simulink model "dual_quaternion_equation_of_motion_1"  (R2016a)
settings: Solver=ode45  StartTime=0.0  StopTime=10.0  MaxStep=0.2  RelTol=1e-3
InitFcn:
  | addpath('..');
settings Model: Creator=AkhramovichSA  LastModifiedBy=AkhramovichSA

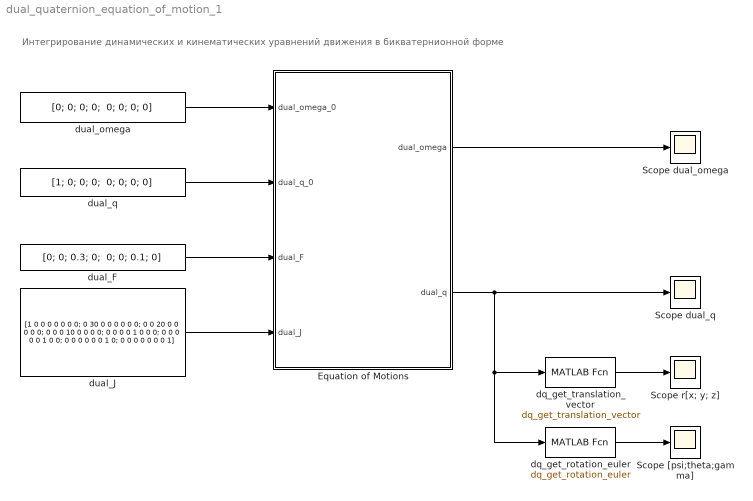
== system dual_quaternion_equation_of_motion_1 ==
  note: Интегрирование динамических и кинематических уравнений движения в бикватернионной форме
  Equation of Motions : Subsystem
  Scope [psi;theta;gamma] : Scope
  Scope dual_omega : Scope
  Scope dual_q : Scope
  Scope r[x; y; z] : Scope
  dq_get_rotation_euler : MATLABFcn  Description=aa  MATLABFcn=dq_get_rotation_euler
  dq_get_translation_vector : MATLABFcn  MATLABFcn=dq_get_translation_vector
  dual_F : Constant  Value="[0; 0; 0.3; 0;  0; 0; 0.1; 0]"  VectorParams1D=off
  dual_J : Constant  Value=[1 0 0 0 0 0 0 0; 0 30 0 0 0 0 0 0; 0 0 20 0 0 0 0 0; 0 0 0 10 0 0 0 0; 0 0 0 0 1 0 0 0; 0 0 0 0 0 1 0 0; 0 0 0 0 0 0 1 0; 0 0 0 0 0 0 0 1]  VectorParams1D=off
  dual_omega : Constant  Value="[0; 0; 0; 0;  0; 0; 0; 0]"  VectorParams1D=off
  dual_q : Constant  Value="[1; 0; 0; 0;  0; 0; 0; 0]"  VectorParams1D=off
  wires:
  dual_J/1 -> Equation of Motions/4(dual_J)
  dual_F/1 -> Equation of Motions/3(dual_F)
  dual_omega/1 -> Equation of Motions/1(dual_omega_0)
  dual_q/1 -> Equation of Motions/2(dual_q_0)
  Equation of Motions/1(dual_omega) -> Scope dual_omega/1
  Equation of Motions/2(dual_q) -> dq_get_rotation_euler/1, dq_get_translation_vector/1, Scope dual_q/1
  dq_get_translation_vector/1 -> Scope r[x; y; z]/1
  dq_get_rotation_euler/1 -> Scope [psi;theta;gamma]/1

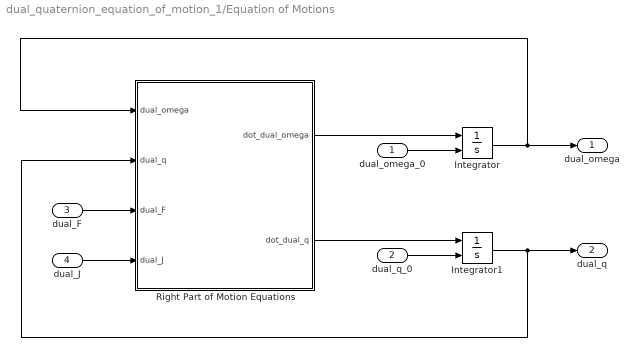
== system dual_quaternion_equation_of_motion_1/Equation of Motions ==
  dual_omega_0 : Inport
  dual_q_0 : Inport  Port=2
  dual_F : Inport  Port=3
  dual_J : Inport  Port=4
  Integrator : Integrator  InitialConditionSource=external
  Integrator1 : Integrator  InitialConditionSource=external
  Right Part of Motion Equations : MATLAB Function  TreatAsAtomicUnit=on
  dual_omega : Outport
  dual_q : Outport  Port=2
  wires:
  Integrator/1 -> dual_omega/1, Right Part of Motion Equations/1(dual_omega)
  dual_omega_0/1 -> Integrator/2
  dual_q_0/1 -> Integrator1/2
  Right Part of Motion Equations/1(dot_dual_omega) -> Integrator/1
  Integrator1/1 -> dual_q/1, Right Part of Motion Equations/2(dual_q)
  Right Part of Motion Equations/2(dot_dual_q) -> Integrator1/1
  dual_F/1 -> Right Part of Motion Equations/3(dual_F)
  dual_J/1 -> Right Part of Motion Equations/4(dual_J)

== matlab function dual_quaternion_equation_of_motion_1/Equation of Motions/Right Part of Motion Equations ==
  data: dual_omega input; dot_dual_omega output; dual_q input; dot_dual_q output; dual_F input; dual_J input
function [dot_dual_omega, dot_dual_q] = dot_dual_omega_q(dual_omega, dual_q, dual_F,  dual_J)
% Правые части динамического и кинематического уравнений движения в бикватернионной форме
% Выходные данные надо проинтегрировать звеном: 1/s

% Входные данные:
%
% Бикватернион угловых и линейных скоростей
% dual_omega = [0; omega_x; omega_y; omega_z; 0; v_x; v_y; v_z]
%
% Бикватернион углового и линейного положения
% dual_q     = [q1; q2; q3; q4; q5; q6; q7; q8]
% 
% Бикватернион моментов и сил
% dual_F     = [0; Mx; My; Mz; 0; Fx; Fy; Fz]
%
% Расширенный тензор инерции в бикватернионной форме
% dual_J     = [1  0   0   0  0  0  0  0;
%               0 Jxx Jxy Jxz 0  0  0  0;
%               0 Jyx Jyy Jyz 0  0  0  0;
%               0 Jzx Jzy Jzz 0  0  0  0;
%               0  0   0   0  1  0  0  0;
%               0  0   0   0  0  m  0  0;
%               0  0   0   0  0  0  m  0;
%               0  0   0   0  0  0  0  m]
% 
% Выходные данные:
% 
% Правая часть дифференциального уравнения динамики, изменение бикватерниона угловых и линейных скоростей
% dot_dual_omega = [0; omega_x; omega_y; omega_z; 0; v_x; v_y; v_z]
%
% Правая часть дифференциального уравнения кинематики, изменение бикватерниона углового и линейного положения
% dot_dual_q     = [q1; q2; q3; q4; q5; q6; q7; q8]

dot_dual_omega = dual_J \ (dual_F - dq_cross([dual_omega(1:4); 0; 0; 0; 0], (dual_J*dual_omega))); 

dot_dual_q     = 0.5*dq_multiply(dual_q, dual_omega);
